simulink model "euler_RBD_together"  (R2019a)
settings: Solver=ode45  StartTime=0.0  StopTime=1000  RelTol=1e-3  EnableMultiTasking=on
settings Model: Creator=Frances  LastModifiedBy=frankiezoo
settings DataIOCC: LimitDataPoints=on  SaveFormat=Array  SignalLoggingSaveFormat=ModelDataLogs  ReturnWorkspaceOutputs=off
settings OptimizationCC: ExpressionDepthLimit=2147483647  LifeSpan=inf
settings DebuggingCC: UnderspecifiedInitializationDetection=Classic  MergeDetectMultiDrivingBlocksExec=none  SolverPrmCheckMsg=warning  FcnCallInpInsideContextMsg=warning  StateNameClashWarn=warning  SFUnexpectedBacktrackingDiag=warning  SFNoUnconditionalDefaultTransitionDiag=warning  SFExecutionAtInitializationDiag=none  ArithmeticOperatorsInVariantConditions=warning
settings HardwareCC: ProdBitPerPointer=32  ProdBitPerSizeT=32  ProdBitPerPtrDiffT=32  ProdLargestAtomicFloat=None  ProdIntDivRoundTo=Undefined  ProdEndianess=Unspecified  ProdWordSize=32  ProdHWDeviceType=32-bit Generic
settings ModelReferenceCC: PropagateSignalLabelsOutOfModel=off
settings SFSimCC: SimUseLocalCustomCode=off  SimParseCustomCode=off
settings RTWCC: RTWUseLocalCustomCode=off
settings CodeAppCC: StateflowObjectComments=on
settings GRTTargetCC: TargetLangStandard=C89/C90 (ANSI)  GeneratePreprocessorConditionals=Disable all  CombineOutputUpdateFcns=off  GRTInterface=on
settings ConfigComp: CovMetricSettings=dw  CovHtmlReporting=on  CovSaveCumulativeToWorkspaceVar=on  CovSaveSingleToWorkspaceVar=on  CovExternalEMLEnable=off

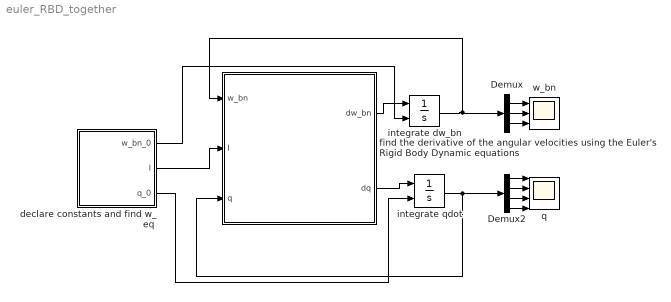
== system euler_RBD_together ==
  Demux : Demux  Outputs=3
  Demux2 : Demux
  declare constants and find w_eq : MATLAB Function  TreatAsAtomicUnit=on
  find the derivative of the angular velocities using the Euler's Rigid Body Dynamic equations : MATLAB Function  TreatAsAtomicUnit=on
  integrate dw_bn : Integrator  InitialConditionSource=external
  integrate qdot : Integrator  InitialConditionSource=external  InitialCondition=[0;0;0;1]
  q : Scope  NumInputPorts=4
  w_bn : Scope  NumInputPorts=3
  wires:
  declare constants and find w_eq/1(w_bn_0) -> integrate dw_bn/2
  find the derivative of the angular velocities using the Euler's Rigid Body Dynamic equations/1(dw_bn) -> integrate dw_bn/1
  Demux/1 -> w_bn/1
  Demux/2 -> w_bn/2
  Demux/3 -> w_bn/3
  integrate qdot/1 -> find the derivative of the angular velocities using the Euler's Rigid Body Dynamic equations/3(q), Demux2/1
  Demux2/1 -> q/1
  Demux2/2 -> q/2
  Demux2/3 -> q/3
  Demux2/4 -> q/4
  integrate dw_bn/1 -> Demux/1, find the derivative of the angular velocities using the Euler's Rigid Body Dynamic equations/1(w_bn)
  declare constants and find w_eq/2(I) -> find the derivative of the angular velocities using the Euler's Rigid Body Dynamic equations/2(I)
  find the derivative of the angular velocities using the Euler's Rigid Body Dynamic equations/2(dq) -> integrate qdot/1
  declare constants and find w_eq/3(q_0) -> integrate qdot/2

== matlab function euler_RBD_together/find the derivative of the angular velocities using the Euler's Rigid Body Dynamic equations ==
  data: w_bn input; dw_bn output; I input; q input; dq output
function [dw_bn,dq]  = plant(w_bn,I,q)
%#eml

qcrs=[q(4) -q(3) q(2)
      q(3) q(4) -q(1)
      -q(2) q(1) q(4)
      -q(1) -q(2) -q(3)];
dq=1/2*qcrs*w_bn;

dw_bn=-inv(I)*(crs(w_bn)*I*w_bn);

end

function [wcrs] = crs(w)
       %Turn a post-multiplying 3x1 vector into a pre-multiplying 3x6 for a symmetric 3x3 matrix.
       wcrs=[ 0    -w(3)  w(2)
              w(3)  0    -w(1)
             -w(2)  w(1)  0   ];
end

== matlab function euler_RBD_together/declare constants and find w_eq ==
  data: w_bn_0 output; I output; q_0 output
function [w_bn_0,I,q_0] = init()
%#eml

m = 1.33 % kg
l = 0.1 % m
I_xx = 1/12*m*(2*l^2) % kg m^2
I_yy = 1/12*m*(2*l^2) % kg m^2
I_zz = 1/12*m*(2*l^2) % kg m^2
I = [I_xx 0 0; 0 I_yy 0; 0 0 I_zz];

w_bn_0=[10;0;0]*pi/180;

phi = pi/4      % "roll" FEEL FREE TO CHANGE THIS VALUE
theta = pi/4       % "pitch" FEEL FREE TO CHANGE THIS VALUE
psi = pi/4      % "yaw" FEEL FREE TO CHANGE THIS VALUE
% rotation matrix 
A_x = [1, 0, 0; 0, cos(phi), -sin(phi);0, sin(phi), cos(phi)];
A_y = [cos(theta), 0, sin(theta); 0, 1, 0; -sin(theta), 0, cos(theta)]
A_z = [cos(psi), -sin(psi), 0; sin(psi), cos(psi), 0;0, 0, 1]
A = A_z * A_y * A_x
% euler axis angle
theta_a = acos((A(1,1)+A(2,2)+A(3,3)-1)/2)
e_1 = (A(3,2)-A(2,3))/(2*sin(theta_a))
e_2 = (A(1,3)-A(3,1))/(2*sin(theta_a))
e_3 = (A(2,1)-A(1,2))/(2*sin(theta_a))
% quaternion
q_x0 = e_1*sin(theta_a/2)
q_y0 = e_2*sin(theta_a/2)
q_z0 = e_3*sin(theta_a/2)
q_w0 = cos(theta_a/2)
q_0 = [q_x0, q_y0, q_z0, q_w0]
